simulink model "sim_topic2"  (R2023b)
settings: Solver=FixedStepAuto  StartTime=0.0  StopTime=T_sim  FixedStep=dt_sim  RelTol=1e-3
undefined symbols (not defined in the file): T
settings Model: Creator=user  LastModifiedBy=user

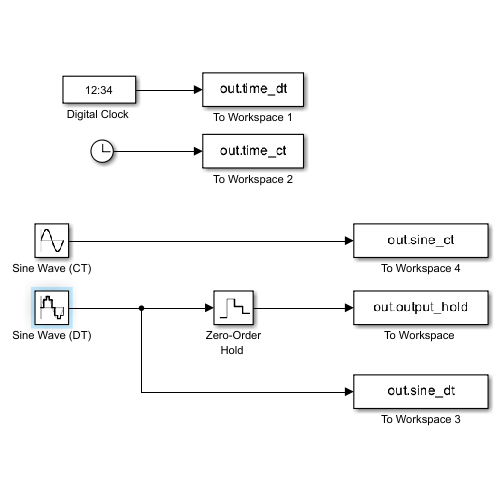
[thumbnail: Simulink's stored preview of the top-level diagram]
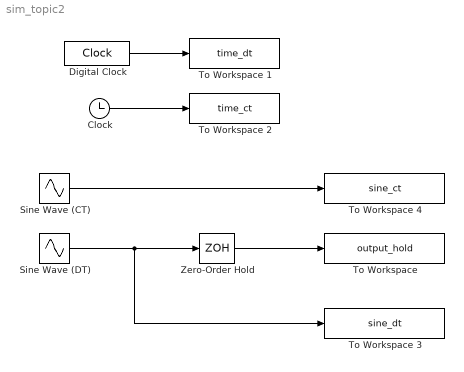
== system sim_topic2 ==
  Clock : Clock
  "Digital Clock " : DigitalClock  SampleTime=T
  Sine Wave (CT) : Sin  Amplitude=3  Frequency=2*pi  SampleTime=0
  Sine Wave (DT) : Sin  Amplitude=3  Frequency=2*pi  SampleTime=T
  "To Workspace " : ToWorkspace  VariableName=output_hold
  To Workspace 1 : ToWorkspace  VariableName=time_dt  SampleTime=T
  To Workspace 2 : ToWorkspace  VariableName=time_ct  SampleTime=-1
  To Workspace 3 : ToWorkspace  VariableName=sine_dt  SampleTime=T
  To Workspace 4 : ToWorkspace  VariableName=sine_ct
  "Zero-Order Hold " : ZeroOrderHold  SampleTime=-1
  wires:
  "Digital Clock "/1 -> To Workspace 1/1
  Clock/1 -> To Workspace 2/1
  Sine Wave (CT)/1 -> To Workspace 4/1
  Sine Wave (DT)/1 -> "Zero-Order Hold "/1, To Workspace 3/1
  "Zero-Order Hold "/1 -> "To Workspace "/1
